simulink model "Biquad_Test_Model"  (R2019b)
settings: Solver=VariableStepAuto  StartTime=0.0  StopTime=testtime  RelTol=1e-3
InitFcn:
  | Biquad_Test_Parameters
StopFcn:
  | Verify_Biquad_Test_Filter
values from neighbouring files (symbols this model uses):
  c1LPihc = ( C - TWOPI*Fcihc ) / ( C + TWOPI*Fcihc )    (= 0.671752219322)    [Biquad_Test_Parameters.m]
  c2LPihc = TWOPI*Fcihc / (TWOPI*Fcihc + C)    (= 0.164123890339)    [Biquad_Test_Parameters.m]
  Fs = 48e3    (= 48000)    [Biquad_Test_Parameters.m]
  gainihc = 1.0    (= 1)    [Biquad_Test_Parameters.m]
undefined symbols (not defined in the file or in its folder): dfilt
libraries: dsparch4 x2, dspsrcs4 x1
settings Model: Creator=mblun  LastModifiedBy=cb50701
settings OptimizationCC: BlockReduction=off  ConditionallyExecuteInputs=off  DefaultParameterBehavior=Inlined
settings DebuggingCC: AlgebraicLoopMsg=error
settings HardwareCC: ProdBitPerPointer=32  ProdBitPerSizeT=32  ProdBitPerPtrDiffT=32  ProdLargestAtomicFloat=None  ProdIntDivRoundTo=Undefined  ProdEndianess=Unspecified  ProdWordSize=32  ProdHWDeviceType=ASIC/FPGA->ASIC/FPGA  TargetBitPerLong=64  TargetBitPerPointer=64  TargetBitPerSizeT=64  TargetBitPerPtrDiffT=64  TargetLongLongMode=on  TargetIntDivRoundTo=Zero  TargetEndianess=LittleEndian  TargetWordSize=64  TargetHWDeviceType=Custom Processor->MATLAB Host Computer  ProdEqTarget=off
settings SFSimCC: CustomCodeUndefinedFunction=UseInterfaceOnly

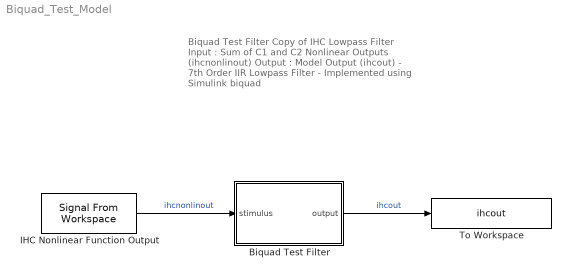
== system Biquad_Test_Model ==
  note: Biquad Test Filter
      | Copy of IHC Lowpass Filter
      |
      | Input : Sum of C1 and C2 Nonlinear Outputs (ihcnonlinout)
      |
      | Output : Model Output (ihcout)
      |
      | - 7th Order IIR Lowpass Filter
      |
      | - Implemented using Simulink biquad
  Biquad Test Filter : Subsystem
  IHC Nonlinear Function Output : dspsrcs4/Signal From Workspace  X=RxSignal  Ts=1/Fs  nsamps=1  OutputAfterFinalValue=Setting to zero  ignoreOrWarnInputAndFrameLengths=off  OutputFrames=off
  To Workspace : ToWorkspace  VariableName=ihcout  SampleTime=-1
      settings: Save2DSignal=2-D array (concatenate along first dimension)
  wires:
  Biquad Test Filter/1(output) -> To Workspace/1  "ihcout"
  IHC Nonlinear Function Output/1 -> Biquad Test Filter/1(stimulus)  "ihcnonlinout"

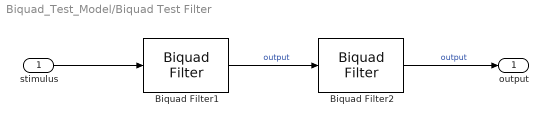
== system Biquad_Test_Model/Biquad Test Filter ==
  stimulus : Inport
  Biquad Filter1 : dsparch4/Biquad Filter  FilterSource=Dialog parameters  CoeffSource=Specify via dialog  FilterObject=dfilt.df2tsos([1 0.3 0.4],[1 0.1 0.2])  IIRFiltStruct=Direct form II transposed  BiQuadCoeffs=[gainihc*c2LPihc gainihc*c2LPihc 0 1 -c1LPihc 0; c2LPihc c2LPihc 0 1 -c1LPihc 0; c2LPihc c2LPihc 0 1 -c1LPihc 0;c2LPihc c2LPihc 0 1 -c1LPihc 0]  ScaleValues=1  IC=0  ICnum=0  ICden=0  a0Flag=Warning  optimizeScaleValues=on  ScaleValueMode=Specify via input port (g)  roundingMode=Floor  overflowMode=on  scaleValueFracLength=14  denProdOutputFracLength=30  denAccumFracLength=30  secondMemoryFracLength=15
      settings: SourceProductName=DSP System Toolbox
  Biquad Filter2 : dsparch4/Biquad Filter  FilterSource=Dialog parameters  CoeffSource=Specify via dialog  FilterObject=dfilt.df2tsos([1 0.3 0.4],[1 0.1 0.2])  IIRFiltStruct=Direct form II transposed  BiQuadCoeffs=[c2LPihc c2LPihc 0 1 -c1LPihc 0; c2LPihc c2LPihc 0 1 -c1LPihc 0; c2LPihc c2LPihc 0 1 -c1LPihc 0]  ScaleValues=1  IC=0  ICnum=0  ICden=0  a0Flag=Warning  optimizeScaleValues=on  ScaleValueMode=Specify via input port (g)  roundingMode=Floor  overflowMode=on  scaleValueFracLength=14  denProdOutputFracLength=30  denAccumFracLength=30  secondMemoryFracLength=15
      settings: SourceProductName=DSP System Toolbox
  output : Outport  VectorParamsAs1DForOutWhenUnconnected=off
  wires:
  stimulus/1 -> Biquad Filter1/1
  Biquad Filter1/1 -> Biquad Filter2/1  "output"
  Biquad Filter2/1 -> output/1  "output"
